simulink model "train_fuzzy2"  (R2017b)
settings: Solver=FixedStepAuto  StartTime=0.0  StopTime=10  FixedStep=0.01  RelTol=1e-3
libraries: fuzblock x1
settings Model: Creator=QuocViet  LastModifiedBy=DELL
settings DebuggingCC: UnconnectedInputMsg=none  UnconnectedOutputMsg=none  UnconnectedLineMsg=none  SFMachineParentedDataDiag=error
settings SFSimCC: SimUseLocalCustomCode=on
settings RTWCC: RTWUseLocalCustomCode=on

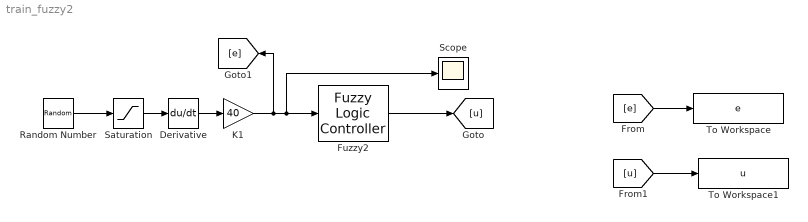
== system train_fuzzy2 ==
  Derivative : Derivative
  Fuzzy2 : fuzblock/Fuzzy Logic  Controller  FIS='RULE222.fis'  OutputSampleNumber=101  DataType=double  FuzzifiedInputs=off  RuleFiringStrengths=off  RuleOutputs=off  AggregatedOutputs=off  SimulateUsing=Interpreted execution
  K1 : Gain  Gain=40
  Random Number : RandomNumber  Variance=pi/2  SampleTime=0.1
  Saturation : Saturate  UpperLimit=pi/2  LowerLimit=-pi/2
  Scope : Scope
  To Workspace : ToWorkspace  VariableName=e  SampleTime=-1
  To Workspace1 : ToWorkspace  VariableName=u  SampleTime=-1
  wires:
  Random Number/1 -> Saturation/1
  K1/1 -> Scope/1, Fuzzy2/1, [e]
  Fuzzy2/1 -> [u]
  Saturation/1 -> Derivative/1
  [e] -> To Workspace/1
  [u] -> To Workspace1/1
  Derivative/1 -> K1/1
